simulink model "HighTemperatureOven_FullStateFeedback_Simulink2019b"  (R2020b)
settings: Solver=ode4  StartTime=0.0  StopTime=SIM_TIME  FixedStep=STEP_SIZE  RelTol=1e-3
undefined symbols (not defined in the file): Cg, Cs, k, kc, Kfs, kg, Ki, kr, t_step_Ta, t_step_Tg, Ta0K, TafK, Tg0K, TgfK, Ts0K, Tsampl, u0, umax, umin, xi0, xss
settings Model: Creator=Mikkel  LastModifiedBy=roga
settings DataIOCC: LimitDataPoints=on  SaveFormat=Array  ReturnWorkspaceOutputs=off
settings OptimizationCC: ExpressionDepthLimit=2147483647  LifeSpan=inf
settings DebuggingCC: UnderspecifiedInitializationDetection=Classic  MergeDetectMultiDrivingBlocksExec=none  SolverPrmCheckMsg=warning  FcnCallInpInsideContextMsg=warning  StateNameClashWarn=warning  SFUnexpectedBacktrackingDiag=warning  SFNoUnconditionalDefaultTransitionDiag=warning  SFExecutionAtInitializationDiag=none  ArithmeticOperatorsInVariantConditions=warning
settings HardwareCC: ProdBitPerPointer=32  ProdBitPerSizeT=32  ProdBitPerPtrDiffT=32  ProdLargestAtomicFloat=None  ProdIntDivRoundTo=Undefined  ProdEndianess=Unspecified  ProdWordSize=32  ProdHWDeviceType=32-bit Generic
settings ModelReferenceCC: PropagateSignalLabelsOutOfModel=off
settings SFSimCC: SimUseLocalCustomCode=off  CustomCodeUndefinedFunction=UseInterfaceOnly
settings RTWCC: RTWUseLocalCustomCode=off
settings CodeAppCC: StateflowObjectComments=on
settings GRTTargetCC: TargetLangStandard=C89/C90 (ANSI)  CombineOutputUpdateFcns=off  GRTInterface=on
settings ConfigComp: CovMetricSettings=dw  CovSaveCumulativeToWorkspaceVar=on  CovSaveSingleToWorkspaceVar=on  CovExternalEMLEnable=off  CovSFcnEnable=off

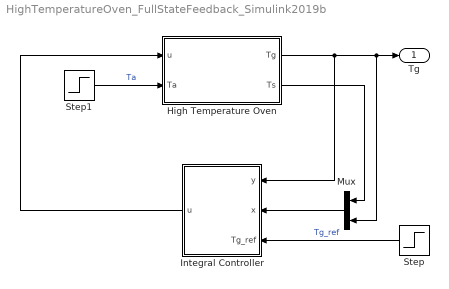
== system HighTemperatureOven_FullStateFeedback_Simulink2019b ==
  High Temperature Oven : Subsystem
  Integral Controller : Subsystem
  Mux : Mux  Inputs=2
  Step : Step  Time=t_step_Tg  Before=Tg0K  After=TgfK  SampleTime=Tsampl
  Step1 : Step  Time=t_step_Ta  Before=Ta0K  After=TafK  SampleTime=0
  Tg : Outport
  wires:
  Step1/1 -> High Temperature Oven/2(Ta)  "Ta"
  High Temperature Oven/1(Tg) -> Integral Controller/1(y), Mux/2, Tg/1
  Step/1 -> Integral Controller/3(Tg_ref)  "Tg_ref"
  Integral Controller/1(u) -> High Temperature Oven/1(u)
  Mux/1 -> Integral Controller/2(x)
  High Temperature Oven/2(Ts) -> Mux/1

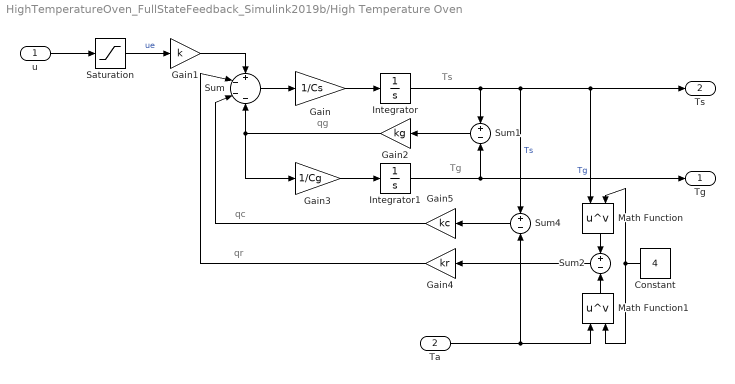
== system HighTemperatureOven_FullStateFeedback_Simulink2019b/High Temperature Oven ==
  note: qg
  note: Ts
  note: Tg
  note: qr
  note: qc
  u : Inport
  Ta : Inport  Port=2
  Constant : Constant  Value=4
  Gain : Gain  Gain=1/Cs
  Gain1 : Gain  Gain=k
  Gain2 : Gain  Gain=kg
  Gain3 : Gain  Gain=1/Cg
  Gain4 : Gain  Gain=kr
  Gain5 : Gain  Gain=kc
  Integrator : Integrator  Priority=1  InitialCondition=Ts0K
  Integrator1 : Integrator  Priority=2  InitialCondition=Tg0K
  Math Function : Math  Operator=pow  SignedPower=on  SaturateOnIntegerOverflow=on
  Math Function1 : Math  Operator=pow  SignedPower=on  SaturateOnIntegerOverflow=on
  Saturation : Saturate  UpperLimit=umax  LowerLimit=umin
  Sum : Sum  Inputs=+---
  Sum1 : Sum  Inputs=+-
  Sum2 : Sum  Inputs=+-
  Sum4 : Sum  Inputs=+-
  Tg : Outport
  Ts : Outport  Port=2
  wires:
  Gain3/1 -> Integrator1/1
  Gain2/1 -> Gain3/1, Sum/4
  Integrator/1 -> Sum1/1, Sum4/1, Ts/1, Math Function/1  "Ts"
  Gain5/1 -> Sum/3
  Math Function1/1 -> Sum2/2
  Ta/1 -> Math Function1/1, Sum4/2
  Constant/1 -> Math Function/2, Math Function1/2
  Gain1/1 -> Sum/1
  Math Function/1 -> Sum2/1
  Sum2/1 -> Gain4/1
  Gain4/1 -> Sum/2
  Sum4/1 -> Gain5/1
  Sum1/1 -> Gain2/1
  Sum/1 -> Gain/1
  Integrator1/1 -> Tg/1, Sum1/2  "Tg"
  Gain/1 -> Integrator/1
  Saturation/1 -> Gain1/1  "ue"
  u/1 -> Saturation/1

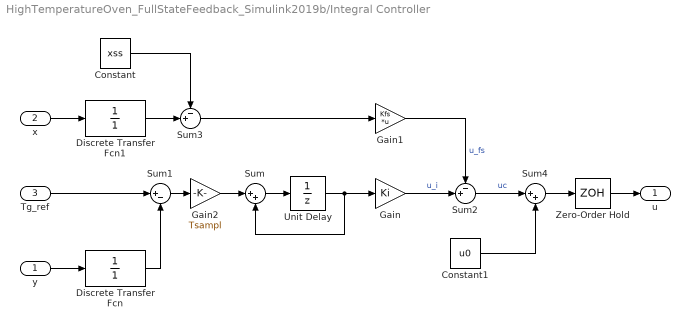
== system HighTemperatureOven_FullStateFeedback_Simulink2019b/Integral Controller ==
  y : Inport
  x : Inport  Port=2
  Tg_ref : Inport  Port=3
  Constant : Constant  Value=xss  SampleTime=Tsampl
  Constant1 : Constant  Value=u0  SampleTime=Tsampl
  Discrete Transfer Fcn : DiscreteTransferFcn  Denominator=[1]  SampleTime=Tsampl
  Discrete Transfer Fcn1 : DiscreteTransferFcn  Denominator=[1]  SampleTime=Tsampl
  Gain : Gain  Gain=Ki
  Gain1 : Gain  Gain=Kfs  Multiplication=Matrix(K*u) (u vector)
  Gain2 : Gain  Gain=Tsampl
  Sum : Sum  Inputs=|++
  Sum1 : Sum  Inputs=|+-
  Sum2 : Sum  Inputs=-+|
  Sum3 : Sum  Inputs=-+|
  Sum4 : Sum  Inputs=|++
  Unit Delay : UnitDelay  InitialCondition=xi0  SampleTime=Tsampl  HasFrameUpgradeWarning=on
  Zero-Order Hold : ZeroOrderHold  SampleTime=Tsampl
  u : Outport
  wires:
  x/1 -> Discrete Transfer Fcn1/1
  Tg_ref/1 -> Sum1/1
  y/1 -> Discrete Transfer Fcn/1
  Sum1/1 -> Gain2/1
  Unit Delay/1 -> Gain/1, Sum/2
  Discrete Transfer Fcn/1 -> Sum1/2
  Gain1/1 -> Sum2/1  "u_fs"
  Sum/1 -> Unit Delay/1
  Gain/1 -> Sum2/2  "u_i"
  Sum3/1 -> Gain1/1
  Discrete Transfer Fcn1/1 -> Sum3/2
  Constant/1 -> Sum3/1
  Gain2/1 -> Sum/1
  Sum2/1 -> Sum4/1  "uc"
  Sum4/1 -> Zero-Order Hold/1
  Constant1/1 -> Sum4/2
  Zero-Order Hold/1 -> u/1
